simulink model "MLIB_MacSat_BAM_F16"  (Simulink 8.3)
settings: Solver=ode45  StartTime=0.0  StopTime=10.0  RelTol=1e-3
settings Model: Creator=RE004C  LastModifiedBy=B17364
settings OptimizationCC: ExpressionDepthLimit=2147483647
settings DebuggingCC: FcnCallInpInsideContextMsg=UseLocalSettings  StrictBusMsg=Warning
settings HardwareCC: ProdLargestAtomicInteger=Long  ProdLargestAtomicFloat=Double  ProdIntDivRoundTo=Zero  ProdEndianess=BigEndian  ProdHWDeviceType=Freescale->32-bit PowerPC

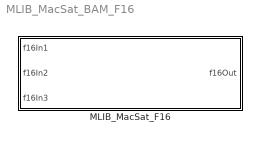
== system MLIB_MacSat_BAM_F16 ==
  MLIB_MacSat_F16 : Subsystem  mask(MLIB_MacSat_F16){}
      mask help: Bit accurate model of saturated multiply-accumulate of input values, staturated if necessary. All parameters as well as input and output are 16bit integers.
      mask init:
      | pos = get_param(gcb, 'Position');width = pos(3) - pos(1); height = pos(4) - pos(2);tX=width/2;tY=height*0.9;
      mask Display: color('black');port_label('input',1,'f16In1');port_label('input',2,'f16In2');port_label('input',3,'f16In3');port_label('output',1,'f16Out');color('black');disp('MLIB_MacSat_F16');color('blue');text(tX,tY, 'BAM', 'horizontalAlignment', 'center');

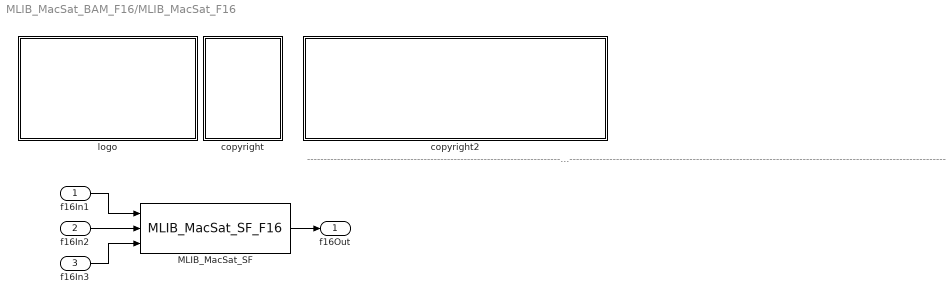
== system MLIB_MacSat_BAM_F16/MLIB_MacSat_F16 ==
  note: ---------------------------------------------------------------------------------------------------------------------------------------------------------------------------------------------------
  f16In1 : Inport
  f16In2 : Inport  Port=2
  f16In3 : Inport  Port=3
  MLIB_MacSat_SF : S-Function  FunctionName=MLIB_MacSat_SF_F16  EnableBusSupport=off
  copyright : Subsystem
      mask Display:
      | text(10,90,'FILE:');text(10,75,'DESRIPTION:')
      | text(10,60,'COPYRIGHT:')
      | text(10,45,'VERSION:')
      | text(10,30,'DATE:')
  copyright2 : Subsystem
      mask Display:
      | text(10,90,'MLIB_MacSat_BAM_F16.mdl');text(10,75,'Saturated sum of two input values.');text(10,60,'Freescale')
      | text(10,45,'0.1');text(10,30,'22-Aug-2011');
  logo : Subsystem
      mask Display: image(imread('logo.jpg'))
  f16Out : Outport
  wires:
  f16In1/1 -> MLIB_MacSat_SF/1
  f16In2/1 -> MLIB_MacSat_SF/2
  f16In3/1 -> MLIB_MacSat_SF/3
  MLIB_MacSat_SF/1 -> f16Out/1

== system MLIB_MacSat_BAM_F16/MLIB_MacSat_F16/copyright ==

== system MLIB_MacSat_BAM_F16/MLIB_MacSat_F16/copyright2 ==

== system MLIB_MacSat_BAM_F16/MLIB_MacSat_F16/logo ==
